simulink model "sampleModel30"  (R2021b)
settings: Solver=VariableStepAuto  StartTime=0.0  StopTime=10.0  RelTol=1e-3
undefined symbols (not defined in the file or in its folder): DiscIntNeverNeededParam
libraries: simulink x6
settings Model: Creator=user  LastModifiedBy=user

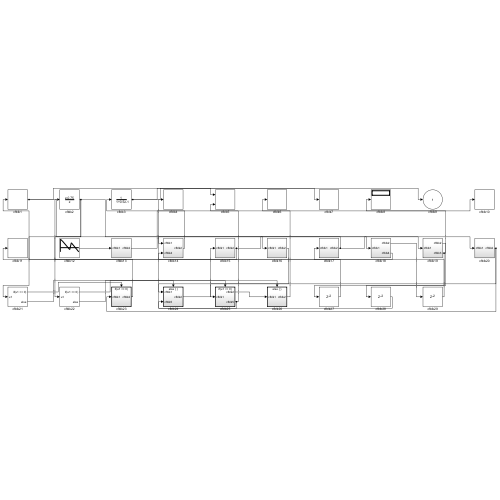
[thumbnail: Simulink's stored preview of the top-level diagram]
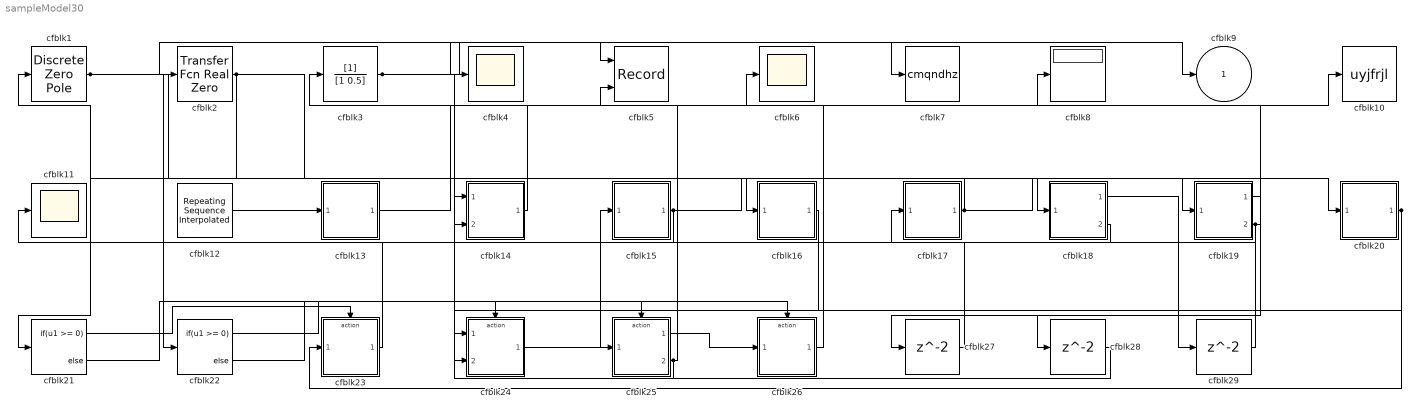
== system sampleModel30 ==
  cfblk1 : DiscreteZeroPole  Poles=[0 0.5]  Gain=1
  cfblk10 : ToWorkspace  VariableName=uyjfrjl  SaveFormat=Timeseries  SampleTime=-1
  cfblk11 : Scope
  cfblk12 : simulink/Sources/Repeating Sequence Interpolated  OutValues=[817556358.798434, 667179918.920058, -217232369.071804, 467958198.571610, -418679929.864932]  TimeValues=[0 0.1 0.5 0.6 1].'  LookUpMeth=Use Input Nearest  tsamp=0.01  OutMin=[]  OutMax=[]  OutDataTypeStr=double  OutputDataTypeScalingMode=double  OutDataType=fixdt(0,8)  OutScaling=2^-10
  cfblk13 : Subsystem
  cfblk14 : Subsystem
  cfblk15 : Subsystem
  cfblk16 : Subsystem
  cfblk17 : Subsystem
  cfblk18 : Subsystem
  cfblk19 : Subsystem
  cfblk2 : simulink/Discrete/Transfer Fcn Real Zero  ZeroZ=0.75  ICPrevInput=0.0  DoSatur=off
      settings: SourceProductBaseCode=SL
  cfblk20 : Subsystem
  cfblk21 : If  IfExpression=u1 >= 0  SampleTime=1
  cfblk22 : If  IfExpression=u1 >= 0  SampleTime=1
  cfblk23 : Subsystem  TreatAsAtomicUnit=on
  cfblk24 : Subsystem  TreatAsAtomicUnit=on
  cfblk25 : Subsystem  TreatAsAtomicUnit=on
  cfblk26 : Subsystem  TreatAsAtomicUnit=on
  cfblk27 : Delay  SampleTime=1
  cfblk28 : Delay  SampleTime=1
  cfblk29 : Delay  SampleTime=1
  cfblk3 : DiscreteFilter  SampleTime=1
  cfblk4 : Scope
  cfblk5 : Record  FileSettingsInternal="{\"entries\":[{\"content\":{\"excelSettings\":{\"content\":{},\"type\":\"Streamout.ExcelSettings\"}},\"type\":\"Streamout.FileSettingStorage\",\"uuid\":\"7cc99ade-53f6-40a6-8694-561096d28d0c\"}],\"packageUris\":[\"http://schema.mathworks.com/mf0/streamout_blocks/R2020a\"],\"version\":\"1.0\"}"  Layout=[1 1]  SignalsInternal="{\"entries\":[{\"content\":{\"signals\":[{\"content\":{\"blockPath\":[\"sampleModel30/cfblk5\"],\"channel\":[],\"dimensions\":[1],\"domain\":\"sampleModel30/cfblk5\",\"lineColor\":\"#a2142f\",\"plots\":[1],\"port\":1,\"sid\":[\"\"],\"signalID\":1157,\"signalName\":\"cfblk1\"},\"type\":\"RecordBlkView.Signal\",\"uuid\":\"ceeb767c-0ab7-4fbb-801a-3501014df9b9\"},{\"content\":{\"blockPath\":[\"sampleModel30/cfblk5\"],\"channel\":[],\"dimensions\":[1],\"domain\":\"sampleModel30/cfblk5\",\"lineColor\":\"#139fff\",\"plots\":[1],\"port\":2,\"sid\":[\"\"],\"signalID\":1161,\"signalName\":\"cfblk25:2\"},\"type\":\"RecordBlkView.Signal\",\"uuid\":\"a3344714-3846-41b3-b737-9db85acf171a\"}]},\"type\":\"RecordBlkView.InputSignals\",\"uuid\":\"d05632e5-c5e0-46ed-b5ca-1da93a2e2e40\"}],\"packageUris\":[\"http://schema.mathworks.com/mf0/streamout_blocks/R2020a\"],\"version\":\"1.0\"}"  VisualizationBindings="{\"xyplotplugin\":{\"info\":[{\"series\":[{\"bindingParametersList\":[{\"parameter\":\"X-Axis\",\"signalID\":1157,\"signalName\":\"cfblk1\"},{\"parameter\":\"Y-Axis\",\"signalID\":1161,\"signalName\":\"cfblk25:2\"}],\"seriesID\":14340}],\"subplotID\":1}]}}"  CompatibilityTag=XY
  cfblk6 : Scope
  cfblk7 : ToWorkspace  VariableName=cmqndhz  SaveFormat=Timeseries  SampleTime=-1
  cfblk8 : Display
  cfblk9 : Outport
  wires:
  cfblk3/1 -> cfblk9/1, cfblk7/1
  cfblk25/1(cfblk2) -> cfblk26/1(cfblk1)
  cfblk25/2(cfblk5) -> cfblk4/1, cfblk5/2
  cfblk12/1 -> cfblk13/1(cfblk1)
  cfblk14/1(cfblk2) -> cfblk3/1
  cfblk1/1 -> cfblk16/1(cfblk1), cfblk5/1
  cfblk2/1 -> cfblk18/1(cfblk1), cfblk22/1, cfblk21/1
  cfblk17/1(cfblk2) -> cfblk14/1(cfblk1), cfblk20/1(cfblk1)
  cfblk16/1(cfblk2) -> cfblk24/1(cfblk1)
  cfblk23/1(cfblk2) -> cfblk11/1
  cfblk13/1(cfblk2) -> cfblk10/1
  cfblk20/1(cfblk2) -> cfblk23/1(cfblk1), cfblk25/1(cfblk1)
  cfblk26/1(cfblk2) -> cfblk6/1
  cfblk24/1(cfblk2) -> cfblk15/1(cfblk1)
  cfblk15/1(cfblk2) -> cfblk19/1(cfblk1), cfblk14/2(cfblk4)
  cfblk18/2(cfblk4) -> cfblk17/1(cfblk1)
  cfblk19/2(cfblk3) -> cfblk8/1, cfblk28/1
  cfblk21/1 -> cfblk23/Action
  cfblk21/2 -> cfblk24/Action
  cfblk22/1 -> cfblk25/Action
  cfblk22/2 -> cfblk26/Action
  cfblk19/1(cfblk2) -> cfblk27/1
  cfblk27/1 -> cfblk1/1
  cfblk28/1 -> cfblk24/2(cfblk5)
  cfblk18/1(cfblk2) -> cfblk29/1
  cfblk29/1 -> cfblk2/1

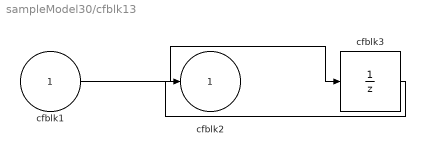
== system sampleModel30/cfblk13 ==
  cfblk1 : Inport
  cfblk3 : UnitDelay  HasFrameUpgradeWarning=on
  cfblk2 : Outport
  wires:
  cfblk1/1 -> cfblk3/1
  cfblk3/1 -> cfblk2/1

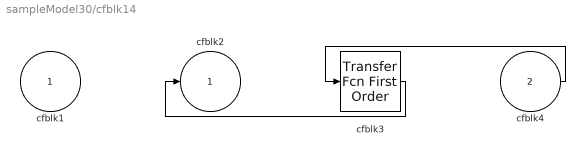
== system sampleModel30/cfblk14 ==
  cfblk1 : Inport
  cfblk4 : Inport  Port=2
  cfblk3 : simulink/Discrete/Transfer Fcn First Order  PoleZ=0.95  ICPrevOutput=0.0  DoSatur=off
  cfblk2 : Outport
  wires:
  cfblk4/1 -> cfblk3/1
  cfblk3/1 -> cfblk2/1

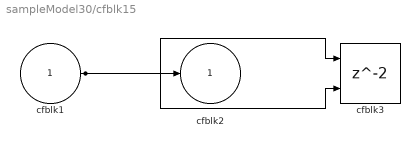
== system sampleModel30/cfblk15 ==
  cfblk1 : Inport
  cfblk3 : Delay  ShowEnablePort=on  SampleTime=1
      settings: InputPortMap=u0,e6
  cfblk2 : Outport
  wires:
  cfblk1/1 -> cfblk2/1, cfblk3/1, cfblk3/2

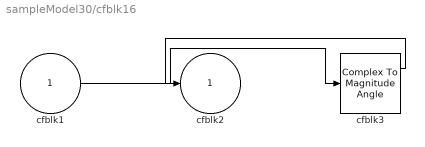
== system sampleModel30/cfblk16 ==
  cfblk1 : Inport
  cfblk3 : ComplexToMagnitudeAngle
  cfblk2 : Outport
  wires:
  cfblk1/1 -> cfblk3/1
  cfblk3/1 -> cfblk2/1

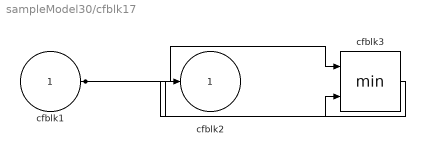
== system sampleModel30/cfblk17 ==
  cfblk1 : Inport
  cfblk3 : MinMax  Inputs=2
  cfblk2 : Outport
  wires:
  cfblk1/1 -> cfblk3/1, cfblk3/2
  cfblk3/1 -> cfblk2/1

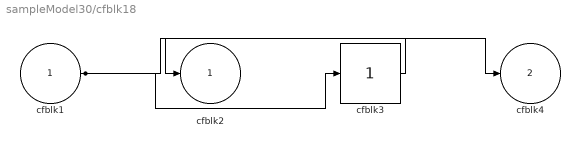
== system sampleModel30/cfblk18 ==
  cfblk1 : Inport
  cfblk3 : simulink/Math Operations/Slider Gain  gain=1  low=0  high=2
  cfblk2 : Outport
  cfblk4 : Outport  Port=2
  wires:
  cfblk3/1 -> cfblk2/1
  cfblk1/1 -> cfblk3/1, cfblk4/1

== system sampleModel30/cfblk19 ==
  cfblk1 : Inport
  cfblk2 : Outport
  cfblk3 : Outport  Port=2
  wires:
  cfblk1/1 -> cfblk2/1, cfblk3/1

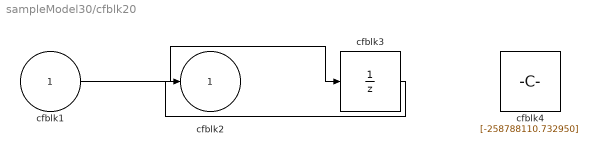
== system sampleModel30/cfblk20 ==
  cfblk1 : Inport
  cfblk3 : UnitDelay  HasFrameUpgradeWarning=on
  cfblk4 : Constant  Value=[-258788110.732950]  SampleTime=1
  cfblk2 : Outport
  wires:
  cfblk1/1 -> cfblk3/1
  cfblk3/1 -> cfblk2/1

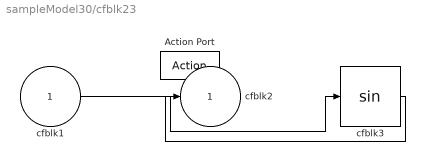
== system sampleModel30/cfblk23 ==
  cfblk1 : Inport
  Action Port : ActionPort  ActionPortLabel=if(u1 >= 0)
  cfblk3 : Trigonometry
  cfblk2 : Outport
  wires:
  cfblk1/1 -> cfblk3/1
  cfblk3/1 -> cfblk2/1

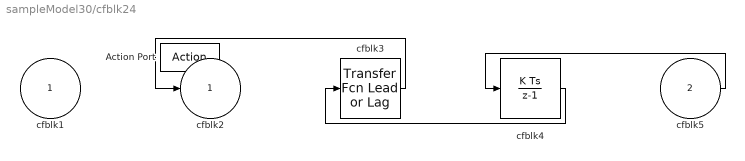
== system sampleModel30/cfblk24 ==
  cfblk1 : Inport
  cfblk5 : Inport  Port=2
  Action Port : ActionPort  ActionPortLabel=else
  cfblk3 : simulink/Discrete/Transfer Fcn Lead or Lag  PoleZ=0.95  ZeroZ=0.75  ICPrevOutput=0.0  ICPrevInput=0.0  DoSatur=off
      settings: SourceProductBaseCode=SL
  cfblk4 : DiscreteIntegrator  SampleTime=-1  ICPrevOutput=DiscIntNeverNeededParam  ICPrevScaledInput=DiscIntNeverNeededParam
  cfblk2 : Outport
  wires:
  cfblk5/1 -> cfblk4/1
  cfblk4/1 -> cfblk3/1
  cfblk3/1 -> cfblk2/1

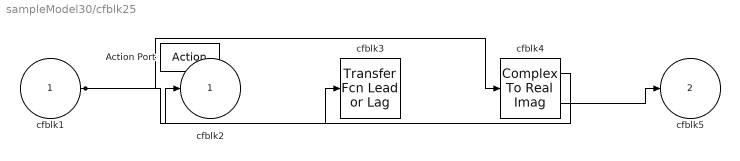
== system sampleModel30/cfblk25 ==
  cfblk1 : Inport
  Action Port : ActionPort  ActionPortLabel=if(u1 >= 0)
  cfblk3 : simulink/Discrete/Transfer Fcn Lead or Lag  PoleZ=0.95  ZeroZ=0.75  ICPrevOutput=0.0  ICPrevInput=0.0  DoSatur=off
      settings: SourceProductBaseCode=SL
  cfblk4 : ComplexToRealImag
  cfblk2 : Outport
  cfblk5 : Outport  Port=2
  wires:
  cfblk4/1 -> cfblk2/1
  cfblk1/1 -> cfblk4/1, cfblk3/1
  cfblk4/2 -> cfblk5/1

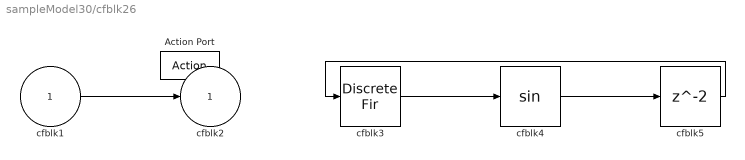
== system sampleModel30/cfblk26 ==
  cfblk1 : Inport
  Action Port : ActionPort  ActionPortLabel=else
  cfblk3 : DiscreteFir
  cfblk4 : Trigonometry
  cfblk5 : Delay
  cfblk2 : Outport
  wires:
  cfblk1/1 -> cfblk2/1
  cfblk3/1 -> cfblk4/1
  cfblk4/1 -> cfblk5/1
  cfblk5/1 -> cfblk3/1
